simulink model "ISC_laboratorio_02_01_02"  (R2019a)
settings: Solver=FixedStepAuto  StartTime=0.0  StopTime=10.0  RelTol=1e-3
undefined symbols (not defined in the file): x0
settings Model: Creator=guilh  LastModifiedBy=guilh
settings DataIOCC: ReturnWorkspaceOutputs=off  TimeSaveName=t

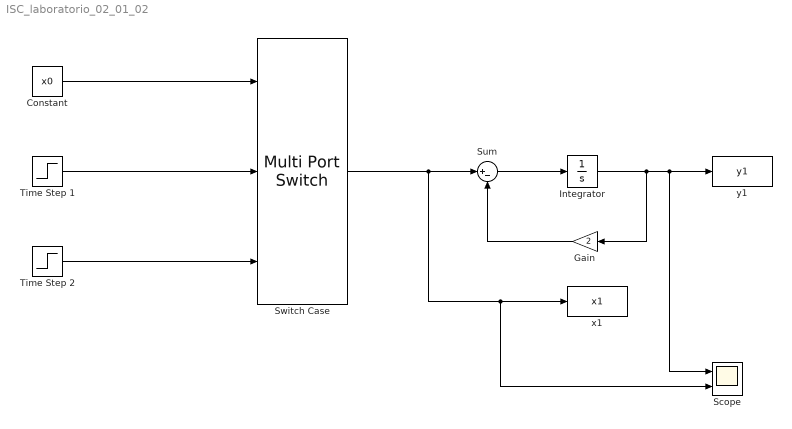
== system ISC_laboratorio_02_01_02 ==
  Constant : Constant  Value=x0
  Gain : Gain  Gain=2
  Integrator : Integrator
  Scope : Scope  NumInputPorts=2
  Sum : Sum  Inputs=|+-
  Switch Case : MultiPortSwitch  Inputs=2
  Time Step 1 : Step  SampleTime=0
  Time Step 2 : Step  Time=2  SampleTime=0
  x1 : ToWorkspace  VariableName=x1  SampleTime=-1
  y1 : ToWorkspace  VariableName=y1  SampleTime=-1
  wires:
  Time Step 2/1 -> Switch Case/3
  Constant/1 -> Switch Case/1
  Integrator/1 -> Gain/1, Scope/1, y1/1
  Sum/1 -> Integrator/1
  Time Step 1/1 -> Switch Case/2
  Switch Case/1 -> Scope/2, x1/1, Sum/1
  Gain/1 -> Sum/2
